simulink model "Bai5B_1"  (R2015a)
settings: Solver=ode45  SolverMode=SingleTasking  StartTime=0.0  StopTime=10.0  RelTol=1e-3
libraries: commfilt2 x2, commchan3 x1, commsink2 x1, commutil2 x1, dspstat3 x1, commanapbnd3 x1, commrandsrc2 x1
settings Model: Creator=MY PC  LastModifiedBy=Ekko
settings OptimizationCC: BlockReduction=off  BooleanDataType=off
settings DebuggingCC: SaveWithParameterizedLinksMsg=none  UnderspecifiedInitializationDetection=Classic  MergeDetectMultiDrivingBlocksExec=none  SignalResolutionControl=TryResolveAllWithWarning
settings HardwareCC: TargetUnknown=on

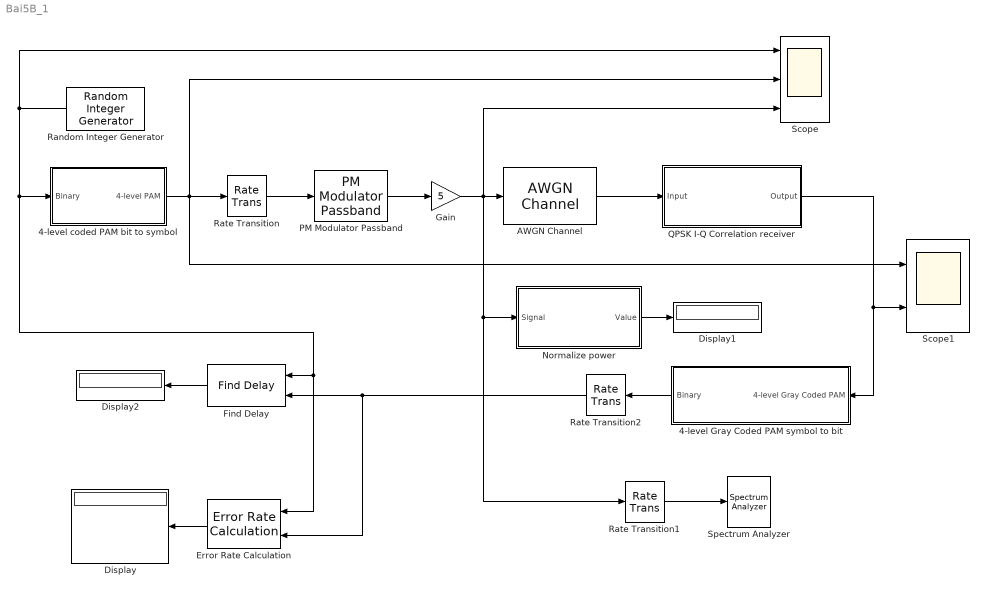
== system Bai5B_1 ==
  4-level Gray Coded PAM symbol to bit : Subsystem
  "4-level coded PAM bit to symbol " : Subsystem
  AWGN Channel : commchan3/AWGN Channel  InputProcessing=Columns as channels (frame based)  seed=67  noiseMode="Signal to noise ratio  (Eb/No)"  EbNodB=10  EsNodB=10  SNRdB=10  bitsPerSym=1  Ps=1  Tsym=1  variance=1
  Display : Display
  Display1 : Display
  Display2 : Display
  Error Rate Calculation : commsink2/Error Rate Calculation  N=0  st_delay=0  cp_mode=Entire frame  subframe=[]  PMode=Port  WsName=ErrorVec  RsMode2=off  stop=off  numErr=100  maxBits=1e6
  Find Delay : commutil2/Find Delay  corrLength=200  chgSigOP=off  stopUpdate=off  numConstDelay=3
  Gain : Gain  Gain=5
  Normalize power : Subsystem
  PM Modulator Passband : commanapbnd3/PM Modulator Passband  Fc=300  Ph=0  Kc=pi/2
  "QPSK I-Q Correlation receiver " : Subsystem
  Random Integer Generator : commrandsrc2/Random Integer Generator  mul=8  seed=37  Ts=1  frameBased=off  sampPerFrame=1  orient=off  outDataType=double
  Rate Transition : RateTransition
  Rate Transition1 : RateTransition  OutPortSampleTime=2e-5
  Rate Transition2 : RateTransition
  Scope : Scope  NumInputPorts=3
      settings: YMin=-5~-5~-5  YMax=5~5~5
  Scope1 : Scope  NumInputPorts=2
      settings: YMin=-5~-5  YMax=5~5
  Spectrum Analyzer : SpectrumAnalyzer
  wires:
  Normalize power/1(Value) -> Display1/1
  Rate Transition1/1 -> Spectrum Analyzer/1
  "4-level coded PAM bit to symbol "/1(4-level PAM) -> Scope1/1, Scope/2, Rate Transition/1
  Rate Transition/1 -> PM Modulator Passband/1
  PM Modulator Passband/1 -> Gain/1
  Gain/1 -> Rate Transition1/1, Normalize power/1(Signal), Scope/3, AWGN Channel/1
  AWGN Channel/1 -> "QPSK I-Q Correlation receiver "/1(Input)
  "QPSK I-Q Correlation receiver "/1(Output) -> 4-level Gray Coded PAM symbol to bit/1("4-level Gray Coded PAM "), Scope1/2
  Random Integer Generator/1 -> Scope/1, Error Rate Calculation/1, Find Delay/1, "4-level coded PAM bit to symbol "/1(Binary)
  4-level Gray Coded PAM symbol to bit/1(Binary) -> Rate Transition2/1
  Rate Transition2/1 -> Error Rate Calculation/2, Find Delay/2
  Find Delay/1 -> Display2/1
  Error Rate Calculation/1 -> Display/1

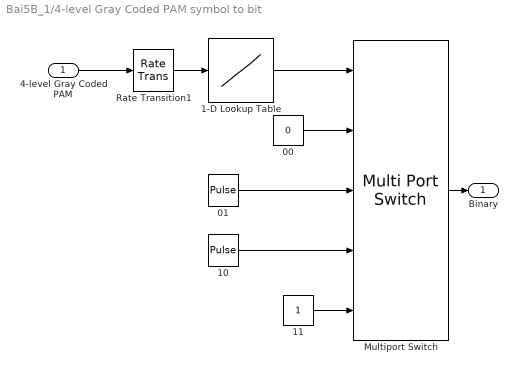
== system Bai5B_1/4-level Gray Coded PAM symbol to bit ==
  "4-level Gray Coded PAM " : Inport
  00 : Constant  Value=0
  "01 " : DiscretePulseGenerator  PulseType=Time based  Period=10  PulseWidth=5
  1-D Lookup Table : Lookup_n-D  NumberOfTableDimensions=1  BreakpointsForDimension1=[-5:5]  Table=tanh([-5:5])  InternalRulePriority=Speed  RndMeth=Simplest  InputSameDT=on
  10 : DiscretePulseGenerator  PulseType=Time based  Period=10  PulseWidth=5
  11 : Constant
  Multiport Switch : MultiPortSwitch  Inputs=4  DiagnosticForDefault=None
  Rate Transition1 : RateTransition
  Binary : Outport
  wires:
  Rate Transition1/1 -> 1-D Lookup Table/1
  11/1 -> Multiport Switch/5
  1-D Lookup Table/1 -> Multiport Switch/1
  "01 "/1 -> Multiport Switch/3
  10/1 -> Multiport Switch/4
  00/1 -> Multiport Switch/2
  Multiport Switch/1 -> Binary/1
  "4-level Gray Coded PAM "/1 -> Rate Transition1/1

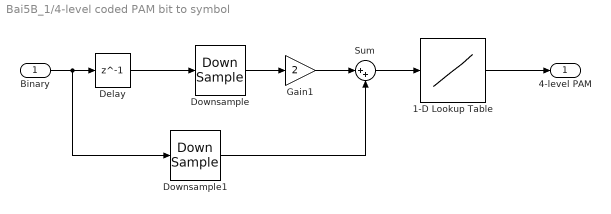
== system Bai5B_1/4-level coded PAM bit to symbol  ==
  Binary : Inport
  1-D Lookup Table : Lookup_n-D  NumberOfTableDimensions=1  BreakpointsForDimension1=[-5:5]  Table=tanh([-5:5])  InternalRulePriority=Speed  RndMeth=Simplest  InputSameDT=on
  Delay : Delay  DelayLength=1  InitialCondition=0
  Downsample : DownSample  RateOptions=Allow multirate processing
  Downsample1 : DownSample  RateOptions=Allow multirate processing
  Gain1 : Gain  Gain=2
  Sum : Sum  Inputs=|++
  4-level PAM : Outport
  wires:
  1-D Lookup Table/1 -> 4-level PAM/1
  Downsample/1 -> Gain1/1
  Delay/1 -> Downsample/1
  Binary/1 -> Downsample1/1, Delay/1
  Downsample1/1 -> Sum/2
  Gain1/1 -> Sum/1
  Sum/1 -> 1-D Lookup Table/1

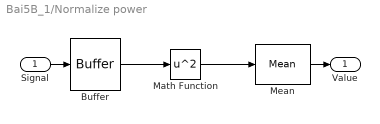
== system Bai5B_1/Normalize power ==
  Signal : Inport
  Buffer : Buffer  TreatMby1Signals=One channel
  Math Function : Math  Operator=square  SaturateOnIntegerOverflow=on
  Mean : dspstat3/Mean  run=off  reset_popup=None  InputProcessing=Columns as channels (frame based)  directionMode=Each column  dimension=1  treatSBRowAsCol=off  roiEnable=off  roiType=Rectangles  roiPortion=Entire ROI  roiOutput=Individual statistics for each ROI  roiFlag=off  outputDataTypeStr=Inherit: Same as accumulator  outputLastDataTypeStr=Inherit: Same as accumulator  outputMin=[]  outputMax=[]  roundingMode=Floor  overflowMode=off
  Value : Outport
  wires:
  Buffer/1 -> Math Function/1
  Signal/1 -> Buffer/1
  Mean/1 -> Value/1
  Math Function/1 -> Mean/1

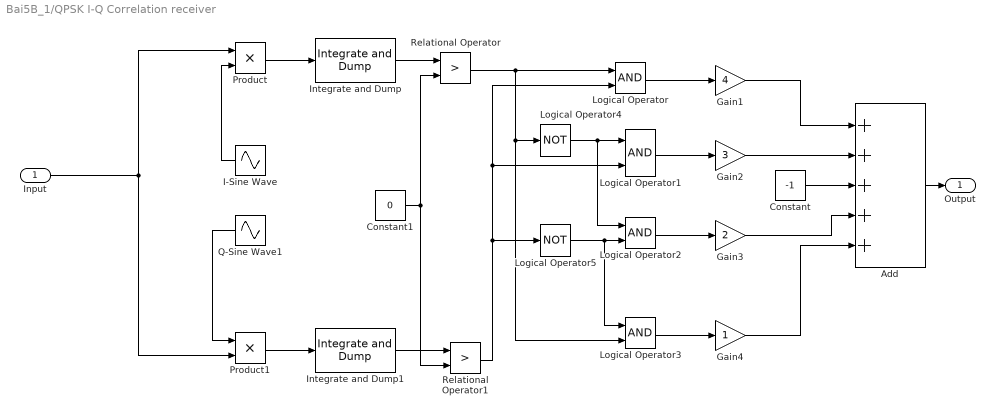
== system Bai5B_1/QPSK I-Q Correlation receiver  ==
  Input : Inport
  Add : Sum  Inputs=+++++
  Constant : Constant  Value=-1
  Constant1 : Constant  Value=0
  Gain1 : Gain  Gain=4
  Gain2 : Gain  Gain=3
  Gain3 : Gain  Gain=2
  Gain4 : Gain
  I-Sine Wave : Sin  Frequency=5000  SampleTime=2e-5
  Integrate and Dump : commfilt2/Integrate and Dump  obssamples=8  offsetsamples=0  nodump=off  roundingMode=Floor  overflowMode=off
  Integrate and Dump1 : commfilt2/Integrate and Dump  obssamples=8  offsetsamples=0  nodump=off  roundingMode=Floor  overflowMode=off
  Logical Operator{,1..3} (4 alike) : Logic  AllPortsSameDT=off  OutDataTypeStr=boolean
  Logical Operator4 : Logic  Operator=NOT  AllPortsSameDT=off  OutDataTypeStr=boolean
  Logical Operator5 : Logic  Operator=NOT  AllPortsSameDT=off  OutDataTypeStr=boolean
  Product : Product
  Product1 : Product
  Q-Sine Wave1 : Sin  Frequency=5000  SampleTime=2e-5
  Relational Operator : RelationalOperator  Operator=>  OutDataTypeStr=boolean
  Relational Operator1 : RelationalOperator  Operator=>  OutDataTypeStr=boolean
  Output : Outport
  wires:
  Add/1 -> Output/1
  Logical Operator2/1 -> Gain3/1
  Logical Operator3/1 -> Gain4/1
  Gain2/1 -> Add/2
  Gain3/1 -> Add/4
  Gain1/1 -> Add/1
  Logical Operator1/1 -> Gain2/1
  Relational Operator1/1 -> Logical Operator5/1, Logical Operator/2, Logical Operator1/2
  Constant/1 -> Add/3
  Gain4/1 -> Add/5
  Logical Operator/1 -> Gain1/1
  Integrate and Dump1/1 -> Relational Operator1/1
  Product/1 -> Integrate and Dump/1
  Integrate and Dump/1 -> Relational Operator/1
  Product1/1 -> Integrate and Dump1/1
  Logical Operator4/1 -> Logical Operator2/1, Logical Operator1/1
  I-Sine Wave/1 -> Product/2
  Logical Operator5/1 -> Logical Operator3/1, Logical Operator2/2
  Relational Operator/1 -> Logical Operator3/2, Logical Operator4/1, Logical Operator/1
  Constant1/1 -> Relational Operator/2, Relational Operator1/2
  Q-Sine Wave1/1 -> Product1/1
  Input/1 -> Product1/2, Product/1
